simulink model "PID_controller_simulation_4"  (Simulink 7.3)
settings: Solver=ode45  StartTime=0.0  StopTime=60  RelTol=1e-3
libraries: powerlib_extras x1, gauges_gmslib x1
settings Model: Creator=cheidelb  LastModifiedBy=STAIB User

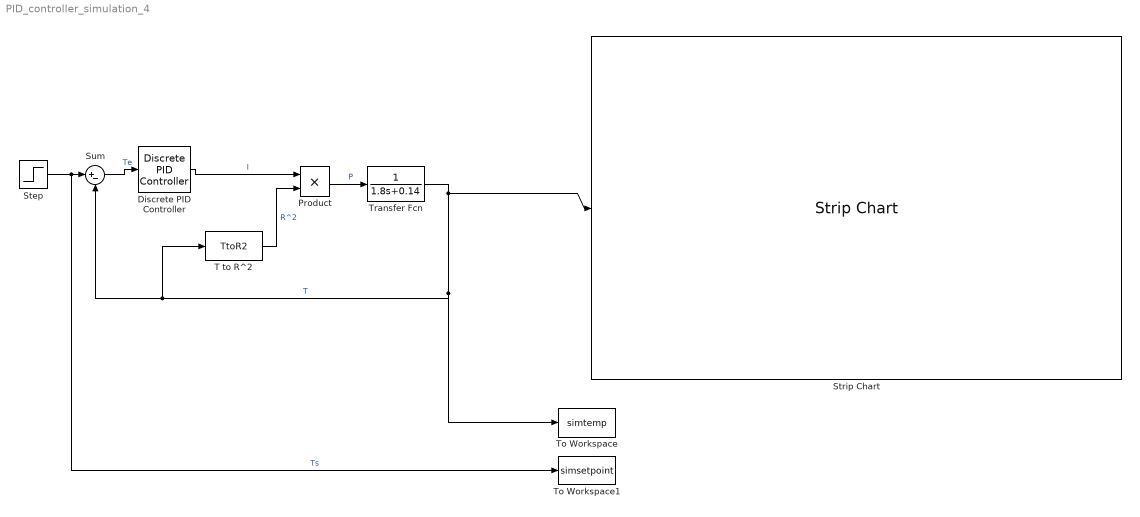
== system PID_controller_simulation_4 ==
  Discrete PID Controller : powerlib_extras/Discrete  Control Blocks/Discrete PID Controller  DialogController=POWERSYS.PowerSysDialog  SystemSampleTime=-1  Kp=.015  Ki=0  Kd=0  TcD=1  Par_Limits=[100 -100]  Init=0  Ts=0.5
  Product : Product  OutDataType=fixdt(1, 16)  OutScaling=2^0  RndMeth=Zero
  Step : Step  Time=20  Before=150  After=500  SampleTime=0
  Strip Chart : gauges_gmslib/Strip Chart/Strip Chart  progid=mwStrip.stripctrl.1  connect=input  init="hActx.XTicMode = 1;hActx.XSpan = 10/60/60/24; hActx.TimeSecondsFormat = '%M:%S'; hActx.TimeDateFormat = ''; hActx.TimeDaysFormat = ''; hActx.TimeHoursFormat = ''; hActx.TimeMinutesFormat = ''; hActx.TimeMonthsFormat = ''; hActx.TimeYearsFormat = ''; % Set x-axis to display time; set span = 10 sec (in fixed units=days); set display format = \"min:sec\" only"  inblock=on  border=on  updateParam=0
  Sum : Sum  Inputs=|+-  OutDataType=fixdt(1, 16)  OutScaling=2^0
  T to R^2 : MATLABFcn  MATLABFcn=TtoR2
  To Workspace : ToWorkspace  VariableName=simtemp  SampleTime=.5  SaveFormat=Structure With Time
  To Workspace1 : ToWorkspace  VariableName=simsetpoint  SampleTime=.5  SaveFormat=Structure With Time
  Transfer Fcn : TransferFcn  Denominator=[1.8 0.14]
  wires:
  T to R^2/1 -> Product/2  "R^2"
  Product/1 -> Transfer Fcn/1  "P"
  Transfer Fcn/1 -> Strip Chart/1, Sum/2, T to R^2/1, To Workspace/1  "T"
  Sum/1 -> Discrete PID Controller/1  "Te"
  Discrete PID Controller/1 -> Product/1  "I"
  Step/1 -> To Workspace1/1, Sum/1  "Ts"
